simulink model "RPP"  (R2023a)
settings: Solver=FixedStepDiscrete  StartTime=0.0  StopTime=10000  FixedStep=Ts_motor  RelTol=1e-3
values from neighbouring files (symbols this model uses):
  desired_linear_vel = 1.0    (= 1)    [init.m]
  goal_dist_tol = 0.05    [init.m]
  L = 0.411    [init.m]
  lookahead_time = 0.55    [init.m]
  max_angular_accel = 4.0    (= 4)    [init.m]
  max_linear_accel = 1.5    [init.m]
  max_linear_decel = 1.5    [init.m]
  max_lookahead_dist = 0.9    [init.m]
  min_lookahead_dist = 0.35    [init.m]
  R = 0.173    [init.m]
  regulated_linear_scaling_min_radius = 0.9    [init.m]
  regulated_linear_scaling_min_speed = 0.2    [init.m]
  rotate_to_heading_angular_vel = 3.0    (= 3)    [init.m]
  theta_0 = atan2(WP(2,2) - WP(1,2), WP(2,1) - WP(1,1))    [run_A_Star.m]
  Ts_motor = 0.05    [init.m]
  WP = [WP; goal_pose]    [run_A_Star.m]
  x_0 = WP(1, 1)    [run_A_Star.m]
  y_0 = WP(1, 2)    [run_A_Star.m]
undefined symbols (not defined in the file or in its folder): den_left, den_right, DiscIntNeverNeededParam, num_left, num_right
settings Model: Creator=HOME  LastModifiedBy=Thu

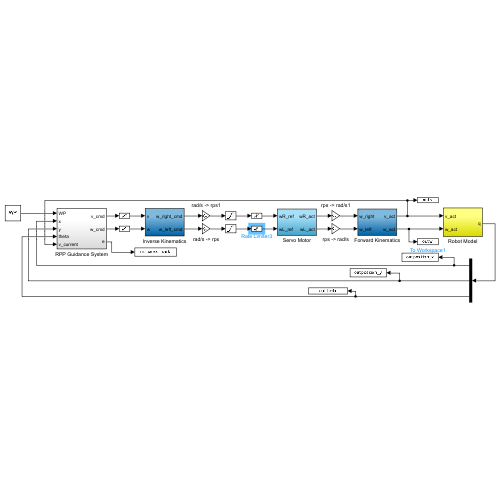
[thumbnail: Simulink's stored preview of the top-level diagram]
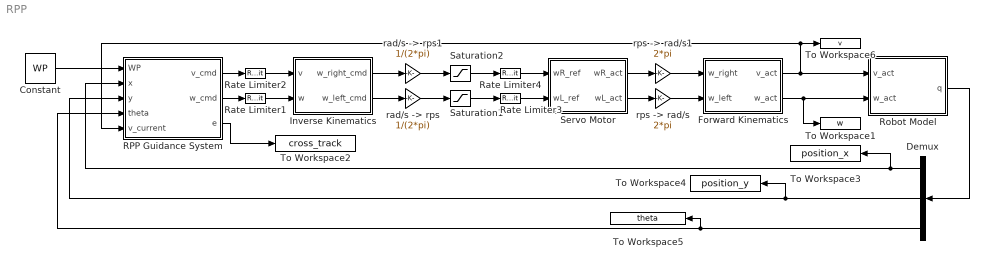
== system RPP ==
  Constant : Constant  Value=WP
  Demux : Demux  Outputs=3
  Forward Kinematics : Subsystem
  Inverse Kinematics : Subsystem
  RPP Guidance System : Subsystem
  Rate Limiter1 : RateLimiter  RisingSlewLimit=max_angular_accel  FallingSlewLimit=-max_angular_accel  SampleTimeMode=inherited
  Rate Limiter2 : RateLimiter  RisingSlewLimit=max_linear_accel  FallingSlewLimit=-max_linear_decel  SampleTimeMode=inherited
  Rate Limiter3 : RateLimiter  RisingSlewLimit=1.5  FallingSlewLimit=-1.5  SampleTimeMode=inherited
  Rate Limiter4 : RateLimiter  RisingSlewLimit=1.5  FallingSlewLimit=-1.5  SampleTimeMode=inherited
  Robot Model : Subsystem
  Saturation1 : Saturate  UpperLimit=2.5  LowerLimit=-2.5
  Saturation2 : Saturate  UpperLimit=2  LowerLimit=-2
  Servo Motor : Subsystem
  To Workspace1 : ToWorkspace  VariableName=w  SampleTime=-1
  To Workspace2 : ToWorkspace  VariableName=cross_track  SampleTime=-1
  To Workspace3 : ToWorkspace  VariableName=position_x  SampleTime=-1
  To Workspace4 : ToWorkspace  VariableName=position_y  SampleTime=-1
  To Workspace5 : ToWorkspace  VariableName=theta  SampleTime=-1
  To Workspace6 : ToWorkspace  VariableName=v  SampleTime=-1
  "rad/s -> rps" : Gain  Gain=1/(2*pi)
  "rad/s -> rps1" : Gain  Gain=1/(2*pi)
  "rps -> rad/s" : Gain  Gain=2*pi
  "rps -> rad/s1" : Gain  Gain=2*pi
  wires:
  Constant/1 -> RPP Guidance System/1(WP)
  Robot Model/1(q) -> Demux/1
  Demux/1 -> To Workspace3/1, RPP Guidance System/2(x)
  Demux/2 -> To Workspace4/1, RPP Guidance System/3(y)
  Demux/3 -> RPP Guidance System/4(theta), To Workspace5/1
  RPP Guidance System/3(e) -> To Workspace2/1
  Forward Kinematics/1(v_act) -> Robot Model/1(v_act), RPP Guidance System/5(v_current), To Workspace6/1
  Forward Kinematics/2(w_act) -> To Workspace1/1, Robot Model/2(w_act)
  RPP Guidance System/1(v_cmd) -> Rate Limiter2/1
  Rate Limiter2/1 -> Inverse Kinematics/1(v)
  Inverse Kinematics/2(w_left_cmd) -> "rad/s -> rps"/1
  "rad/s -> rps"/1 -> Saturation1/1
  "rad/s -> rps1"/1 -> Saturation2/1
  Inverse Kinematics/1(w_right_cmd) -> "rad/s -> rps1"/1
  "rps -> rad/s"/1 -> Forward Kinematics/2(w_left)
  "rps -> rad/s1"/1 -> Forward Kinematics/1(w_right)
  Servo Motor/2(wL_act) -> "rps -> rad/s"/1
  Servo Motor/1(wR_act) -> "rps -> rad/s1"/1
  RPP Guidance System/2(w_cmd) -> Rate Limiter1/1
  Rate Limiter1/1 -> Inverse Kinematics/2(w)
  Saturation1/1 -> Rate Limiter3/1
  Saturation2/1 -> Rate Limiter4/1
  Rate Limiter4/1 -> Servo Motor/1(wR_ref)
  Rate Limiter3/1 -> Servo Motor/2(wL_ref)

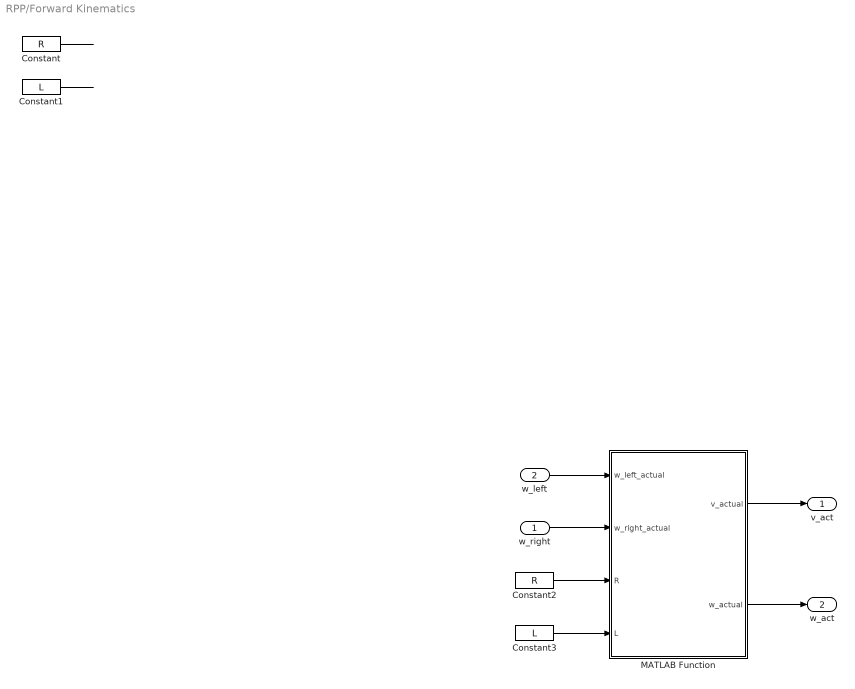
== system RPP/Forward Kinematics ==
  w_right : Inport
  w_left : Inport  Port=2
  Constant : Constant  Value=R
  Constant1 : Constant  Value=L
  Constant2 : Constant  Value=R
  Constant3 : Constant  Value=L
  MATLAB Function : MATLAB Function  TreatAsAtomicUnit=on
  v_act : Outport
  w_act : Outport  Port=2
  wires:
  MATLAB Function/1(v_actual) -> v_act/1
  MATLAB Function/2(w_actual) -> w_act/1
  Constant1/1 -> ?
  Constant/1 -> ?
  Constant3/1 -> MATLAB Function/4(L)
  Constant2/1 -> MATLAB Function/3(R)
  w_right/1 -> MATLAB Function/2(w_right_actual)
  w_left/1 -> MATLAB Function/1(w_left_actual)

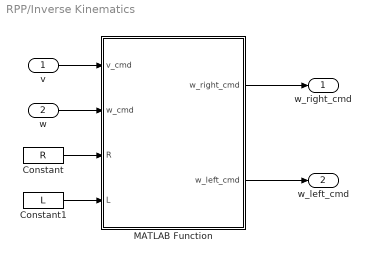
== system RPP/Inverse Kinematics ==
  v : Inport
  w : Inport  Port=2
  Constant : Constant  Value=R
  Constant1 : Constant  Value=L
  MATLAB Function : MATLAB Function  TreatAsAtomicUnit=on
  w_right_cmd : Outport
  w_left_cmd : Outport  Port=2
  wires:
  MATLAB Function/2(w_left_cmd) -> w_left_cmd/1
  MATLAB Function/1(w_right_cmd) -> w_right_cmd/1
  w/1 -> MATLAB Function/2(w_cmd)
  v/1 -> MATLAB Function/1(v_cmd)
  Constant/1 -> MATLAB Function/3(R)
  Constant1/1 -> MATLAB Function/4(L)

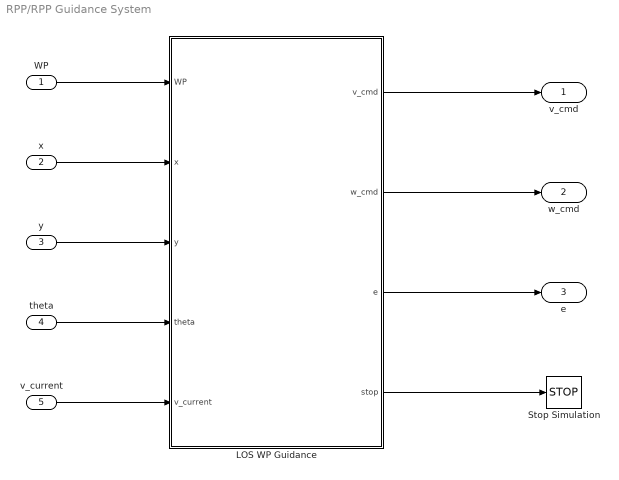
== system RPP/RPP Guidance System ==
  WP : Inport
  x : Inport  Port=2
  y : Inport  Port=3
  theta : Inport  Port=4
  v_current : Inport  Port=5
  "LOS WP Guidance " : MATLAB Function  TreatAsAtomicUnit=on
  Stop Simulation : Stop
  v_cmd : Outport  VectorParamsAs1DForOutWhenUnconnected=off
  w_cmd : Outport  Port=2  VectorParamsAs1DForOutWhenUnconnected=off
  e : Outport  Port=3  VectorParamsAs1DForOutWhenUnconnected=off
  wires:
  y/1 -> "LOS WP Guidance "/3(y)
  "LOS WP Guidance "/4(stop) -> Stop Simulation/1
  x/1 -> "LOS WP Guidance "/2(x)
  WP/1 -> "LOS WP Guidance "/1(WP)
  "LOS WP Guidance "/1(v_cmd) -> v_cmd/1
  "LOS WP Guidance "/3(e) -> e/1
  theta/1 -> "LOS WP Guidance "/4(theta)
  v_current/1 -> "LOS WP Guidance "/5(v_current)
  "LOS WP Guidance "/2(w_cmd) -> w_cmd/1

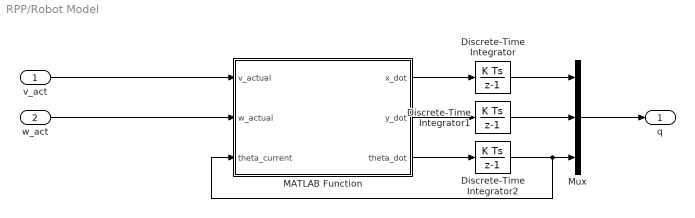
== system RPP/Robot Model ==
  v_act : Inport
  w_act : Inport  Port=2
  Discrete-Time Integrator : DiscreteIntegrator  InitialCondition=x_0  SampleTime=Ts_motor  ICPrevOutput=DiscIntNeverNeededParam  ICPrevScaledInput=DiscIntNeverNeededParam
  Discrete-Time Integrator1 : DiscreteIntegrator  InitialCondition=y_0  SampleTime=Ts_motor  ICPrevOutput=DiscIntNeverNeededParam  ICPrevScaledInput=DiscIntNeverNeededParam
  Discrete-Time Integrator2 : DiscreteIntegrator  InitialCondition=theta_0  SampleTime=Ts_motor  ICPrevOutput=DiscIntNeverNeededParam  ICPrevScaledInput=DiscIntNeverNeededParam
  MATLAB Function : MATLAB Function  TreatAsAtomicUnit=on
  Mux : Mux  Inputs=3
  q : Outport
  wires:
  Discrete-Time Integrator1/1 -> Mux/2
  Mux/1 -> q/1
  Discrete-Time Integrator2/1 -> MATLAB Function/3(theta_current), Mux/3
  Discrete-Time Integrator/1 -> Mux/1
  w_act/1 -> MATLAB Function/2(w_actual)
  v_act/1 -> MATLAB Function/1(v_actual)
  MATLAB Function/1(x_dot) -> Discrete-Time Integrator/1
  MATLAB Function/2(y_dot) -> Discrete-Time Integrator1/1
  MATLAB Function/3(theta_dot) -> Discrete-Time Integrator2/1

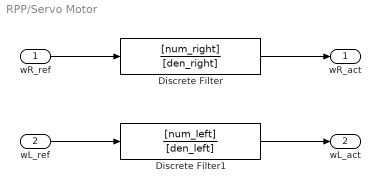
== system RPP/Servo Motor ==
  wR_ref : Inport
  wL_ref : Inport  Port=2
  Discrete Filter : DiscreteFilter  Numerator=[num_right]  Denominator=[den_right]  SampleTime=Ts_motor
  Discrete Filter1 : DiscreteFilter  Numerator=[num_left]  Denominator=[den_left]  SampleTime=Ts_motor
  wR_act : Outport
  wL_act : Outport  Port=2
  wires:
  wL_ref/1 -> Discrete Filter1/1
  wR_ref/1 -> Discrete Filter/1
  Discrete Filter/1 -> wR_act/1
  Discrete Filter1/1 -> wL_act/1

== matlab function RPP/RPP Guidance System/LOS WP Guidance  ==
  settings: updateMethod=DISCRETE
  data: WP input; x input; y input; v_cmd output; w_cmd output; e output; stop output; theta input; v_current input; rotate_to_heading_angular_vel parameter; desired_linear_vel parameter; regulated_linear_scaling_min_speed parameter; lookahead_time parameter; min_lookahead_dist parameter; max_lookahead_dist parameter; regulated_linear_scaling_min_radius parameter; goal_dist_tol parameter
function [v_cmd, w_cmd, e, stop] = RPPGuidance(WP, x, y, theta, v_current, rotate_to_heading_angular_vel, desired_linear_vel, regulated_linear_scaling_min_speed, lookahead_time, min_lookahead_dist, max_lookahead_dist, regulated_linear_scaling_min_radius, goal_dist_tol)
persistent init;
persistent current_wp_index;

%% Initial Parameter's Value
if(isempty(init))
    current_wp_index = 1;
    init    = 1;
end

W_max = rotate_to_heading_angular_vel;
V_max = desired_linear_vel;
V_min = regulated_linear_scaling_min_speed;
lookahead_gain = lookahead_time; 
L_min = min_lookahead_dist;  
L_max = max_lookahead_dist;
r_min = regulated_linear_scaling_min_radius; 
to_goal = goal_dist_tol;

%% Stop Condition
stop = 0;
if current_wp_index >= length(WP(:,1))
    v_cmd = 0;
    w_cmd = 0;
    e     = 0;
    stop  = 1;
    return;
end

%% Calculate RPP Parameter
%  Adaptive Lookahead
L_d = v_current * lookahead_gain;
if L_d < L_min
    L_d = L_min; end
if L_d > L_max
    L_d = L_max; end

%  Find Carrot Point
wp1 = WP(current_wp_index, :);
wp2 = WP(current_wp_index + 1, :);
robot_pos = [x, y]; 
[x_carrot, y_carrot] = findLookaheadPoint(wp1, wp2, robot_pos, L_d);

%  Global to Local Frame
dx = x_carrot - x;
dy = y_carrot - y;
x_local = dx * cos(theta) + dy * sin(theta);    
y_local = -dx * sin(theta) + dy * cos(theta);

%% Calculate Kappa and CTE 
kappa = (2 * y_local) / (L_d^2);
alpha_k = atan2(WP(current_wp_index+1, 2) - WP(current_wp_index,2), WP(current_wp_index+1, 1) - WP(current_wp_index,1));
e = -(x - WP(current_wp_index,1))*sin(alpha_k) + (y - WP(current_wp_index,2))*cos(alpha_k);

%% Heuristics Regulation for v_cmd 
v_cmd = V_max;
if abs(kappa) > (1 / r_min)
    v_cmd = V_max / (r_min * abs(kappa)); 
end

if v_cmd < V_min
    v_cmd = V_min;
end

%% Angular velocity 
w_cmd = v_cmd * kappa;
if w_cmd > W_max
    w_cmd = W_max;
elseif w_cmd < -W_max
    w_cmd = -W_max;
end 

%% Waypoint Switching
dist_to_target = norm(wp2 - robot_pos);
is_last_segment = (current_wp_index == length(WP(:,1)) - 1);
if is_last_segment
    % if last segment, stop when 
    if dist_to_target <= to_goal
        current_wp_index = current_wp_index + 1;
    end
else
    % if not last segment, switch wp: 
    if dist_to_target <= L_d
        current_wp_index = current_wp_index + 1;
    end
end
     
end

function [x_c, y_c] = findLookaheadPoint(wp1, wp2, robot_pos, Ld)
    % wp1 = [x1, y1], wp2 = [x2, y2]
    d = wp2 - wp1;          % Vector hướng của đoạn thẳng
    f = wp1 - robot_pos;    % Vector từ tâm (x,y) robot đến wp1

    a = d * d';
    b = 2 * (f * d');
    c = (f * f') - Ld^2;

    discriminant = b^2 - 4*a*c;
    carrot = [0, 0];
    if discriminant < 0
        carrot = wp2;
    else
        t1 = (-b - sqrt(discriminant)) / (2*a);
        t2 = (-b + sqrt(discriminant)) / (2*a);
        if t2 >= 0 && t2 <= 1
            carrot = wp1 + t2*d;
        elseif t1 >= 0 && t1 <= 1
            carrot = wp1 + t1*d;
        else
            carrot = wp2;
        end
    end
    x_c = carrot(1);
    y_c = carrot(2);
end

== matlab function RPP/Inverse Kinematics/MATLAB Function ==
  data: w_right_cmd output; v_cmd input; w_left_cmd output; w_cmd input; R input; L input
function [w_right_cmd, w_left_cmd] = Inverse_Kinematics(v_cmd, w_cmd, R, L)
    % Đầu vào:
    % v_cmd: Lệnh vận tốc tịnh tiến của xe (m/s)
    % w_cmd: Lệnh vận tốc góc của xe (rad/s)
    % R, L: Thông số cơ khí từ Workspace
    
    % Tính vận tốc dài (m/s) mong muốn cho từng bánh
    v_left  = v_cmd - (w_cmd * L / 2);
    v_right = v_cmd + (w_cmd * L / 2);
    
    % Chuyển từ vận tốc dài (m/s) sang vận tốc góc (rad/s)
    w_left_cmd  = v_left / R;
    w_right_cmd = v_right / R;
end

== matlab function RPP/Robot Model/MATLAB Function ==
  data: v_actual input; x_dot output; w_actual input; theta_current input; y_dot output; theta_dot output
function [x_dot, y_dot, theta_dot] = Robot_Kinematics(v_actual, w_actual, theta_current)
    % Tính vận tốc chiếu lên trục X và Y
    x_dot = v_actual * cos(theta_current);
    y_dot = v_actual * sin(theta_current);
    
    % Vận tốc góc 
    theta_dot = w_actual;
end

== matlab function RPP/Forward Kinematics/MATLAB Function ==
  data: w_left_actual input; v_actual output; w_right_actual input; R input; L input; w_actual output
function [v_actual, w_actual] = Forward_Kinematics(w_left_actual, w_right_actual, R, L)
    v_left  = w_left_actual * R;
    v_right = w_right_actual * R;
    
    v_actual = (v_right + v_left) / 2;
    w_actual = (v_right - v_left) / L;
end
